simulink model "VFlexP_small"  (R2026a)
settings: Solver=ode23tb  StopTime=2  FixedStep=5e-5
model workspace (MAT data in the model file):
  DCop_DCBUCK : object (value not decoded)
  Grid_CCVSC_idx = [2; 3; 4; 5; 6; 7; 8; 9; 10; 11; 12]
  Grid_CCVSCs = 1
  Grid_CCVSCs_buses = 1
  Grid_CCVSCs_toM = [0 1 0 0 0 0 0 0 0 0 0 0 ... (781 elements, 71x11)]
  Grid_C_Lines = 0
  Grid_Cbuses = [0.00666666666667 0.00666666666667]
  Grid_DC : object (value not decoded)
  Grid_DCop_DCBUCK : object (value not decoded)
  Grid_DCop_DC_PES : object (value not decoded)
  Grid_DFIGs = 1
  Grid_DFIGs_buses = 1
  Grid_DGs : string (value not decoded)
  Grid_From_buses = 1
  Grid_GFls = 1
  Grid_GFls_buses = 1
  Grid_GFr_idx = 1
  Grid_GFrs = 1
  Grid_GFrs_buses = 1
  Grid_GFrs_toM = [1; 0]
  Grid_IG_idx = 1
  Grid_IGs = 1
  Grid_IGs_buses = 1
  Grid_IGs_toM = [1; 0; 0]
  Grid_L_Lines = 0.05
  Grid_L_Loads = [0 0]
  Grid_Lines_fromM : object (value not decoded)
  Grid_Lines_toM : object (value not decoded)
  Grid_Load_buses = [1; 2]
  Grid_Load_busesDC = []
  Grid_MSGs = 1
  Grid_MSGs_buses = 1
  Grid_Nbuses = 2
  Grid_PQ_gen = 3
  Grid_Ploads = [0.0075 0.0075]
  Grid_PloadsDC = []
  Grid_Ps_lf = 0.51232912
  Grid_Qloads = [0 0]
  Grid_Qs_lf = -0.00723209333333
  Grid_R_Lines = 0.005
  Grid_R_Loads = [2 2]
  Grid_R_Loads_DC = 0
  Grid_Rcf = [150 150]
  Grid_SCs = 1
  Grid_SCs_buses = 1
  Grid_SG_idx = 1
  Grid_SGs = 1
  Grid_SGs_buses = 1
  Grid_SGs_toM = [1; 0]
  Grid_To_buses = 2
  Grid_VCVSC_idx = [1; 2; 3; 4; 5; 6; 7; 8; 9; 10; 11; 12]
  Grid_VCVSCs = 1
  Grid_VCVSCs_buses = [1; 2; 3; 6; 8; 9; 12; 58; 59; 60; 63; 65]
  Grid_VCVSCs_toM = [1 0 0 0 0 0 0 0 0 0 0 0 ... (852 elements, 71x12)]
  Grid_VSM_idx = 2
  Grid_VSMs = 1
  Grid_VSMs_buses = 1
  Grid_VSMs_toM = [0; 1]
  Grid_admitt_matrix = [2.15353135314-19.7953135314i  -1.9801980198+19.801980198i; -1.9801980198+19.801980198i  2.15353135314-19.7953135314i]
  Grid_admitt_matrix_noloads = [1.98686468647-19.7953135314i  -1.9801980198+19.801980198i; -1.9801980198+19.801980198i  1.98686468647-19.7953135314i]
  Grid_bus = [1; 2]
  Grid_busDC_complexity = 1
  Grid_busDC_complexity_PF = 2
  Grid_bus_complexity = [1 1]
  Grid_bus_complexity_PF = [1 1]
  Grid_buses_lf = 1
  Grid_conductance_matrix = 0.00666666666667
  Grid_conductance_matrix_noloads = 0.00666666666667
  Grid_fref : object (value not decoded)
  Grid_gen_static_params : mBase (value not decoded)
  Grid_iPs_lf = 1.95187031336
  Grid_iQs_lf = -138.272551792
  Grid_iadmitt_matrix = [2.88165849328-0.0982918688642i  2.87905051706-0.123273862303i; 2.87905051706-0.123273862303i  2.88165849328-0.0982918688642i]
  Grid_iadmitt_matrix_noloads = [37.5012524798-37.4874983544i  37.4987475202-37.5125016456i; 37.4987475202-37.5125016456i  37.5012524798-37.4874983544i]
  Grid_iconductance_matrix = 150
  Grid_iconductance_matrix_noloads = 150
  Grid_init_OK_bool = 1
  Grid_intconv_PF : object (value not decoded)
  Grid_lf_op : op_report (value not decoded)
  Grid_lineDC_complexity = []
  Grid_lineDC_complexity_PF = []
  Grid_line_complexity = 1
  Grid_line_complexity_PF = 3
  Grid_loadDC_complexity = []
  Grid_loadDC_complexity_PF = []
  Grid_load_complexity = [3 3]
  Grid_load_complexity_PF = [4 4]
  Grid_opDC_CCVSC : object (value not decoded)
  Grid_opDC_VSM : object (value not decoded)
  Grid_opGFr : object (value not decoded)
  Grid_opVCVSC : object (value not decoded)
  Grid_op_CCVSC : object (value not decoded)
  Grid_op_IG : object (value not decoded)
  Grid_op_SG : object (value not decoded)
  Grid_op_VSM : object (value not decoded)
  Grid_shift_lines = 0
  Grid_tap_lines = 1
  Grid_v_buses_mod = [1 1]
  LinsysParamChangeStruct : Param1 (value not decoded)
  Lline = 0.01
  Rline = 1e-05
  linsys : object (value not decoded)
values from neighbouring files (symbols this model uses):
  block_idx = evalin(mdlWks, [bvarname Generators{i} '_idx'])    [fun_init_units_callback.m]
  Fb = areas    [fun_MATPOWER_to_Excel.m]
  Fi = evalin('base', get_param(block, 'Fi'))    [fun_init_GFr.m]    (also in fun_init_intconv_DC_VSM.m)
  Lf = evalin('base', get_param(block, 'Lf'))    [fun_init_GFr.m]    (also in fun_init_intconv_DC_VSM.m)
  Rf = evalin('base', get_param(block, 'Rf'))    [fun_init_GFr.m]    (also in fun_init_intconv_DC_VSM.m)
symbols that are objects in the model workspace (value not decoded): Grid_DCop_DC_PES, Grid_DCop_DCBUCK, Grid_op_CCVSC, Grid_op_IG, Grid_op_SG, Grid_op_VSM, Grid_opDC_CCVSC, Grid_opDC_VSM, Grid_opGFr, Grid_opVCVSC
undefined symbols (not defined in the file or in its folder): block_buses_DC, CCVSC_idx, Cf, costs, costs2, DFIGs_nodes, DiscIntNeverNeededParam, entity, From_nodes, grid_linsys, Grid_op_DFIG, Grid_op_DFIG_PQ, Grid_op_MSG, Grid_op_SC, Grid_op_VCVSC, Hv, initial_states_grid, Kic, Kiv, Kp_theta, Kp_w, Kpc, Kpv, last_send, Lc, m, Matrix_flux_to_i, mD, mp, MSGs_buses, Nbuses_DC, nq, op_VCVSC, Psche, Rc, rkq1, rkq2, SCs_buses, SCs_nodes, sec_control_structure, set_asked, set_DG_up, set_extra_satur, set_sending_cost, SGs_buses, SGs_nodes, Tf, To_nodes, VI_L, VI_R, WOF_Tf, xkq1, xkq2
libraries: simulink x1045, eeGeneralControl x12, eeTransforms x1, sl_discontinuities x1
(part 9 of 50)

== system VFlexP_small/Grid/Loadflow/Loads/dynamic ==
  v_in_d : Inport
  v_in_q : Inport  Port=2
  Gain1 : Gain  Gain=L_Loads(load_complexity_PF == 1)
  Gain2 : Gain  Gain=R_Loads(load_complexity_PF == 1)
  Gain3 : Gain  Gain=R_Loads(load_complexity_PF == 1)
  Gain4 : Gain  Gain=L_Loads(load_complexity_PF == 1)
  Gain5 : Gain  Gain=omegab./L_Loads(load_complexity_PF == 1)
  Gain7 : Gain  Gain=omegab./L_Loads(load_complexity_PF == 1)
  One : Constant  OutDataTypeStr=Inherit: Inherit via back propagation
  Product : Product
  Product1 : Product
  Selector : Selector  InputPortWidth=length(Load_buses)  IndexOptions=Index vector (dialog)  Indices=find(load_complexity_PF == 1)  OutputSizes=1
  Selector1 : Selector  InputPortWidth=length(Load_buses)  IndexOptions=Index vector (dialog)  Indices=find(load_complexity_PF == 1)  OutputSizes=1
  Sum4 : Sum  Inputs=+-|
  Sum5 : Sum  Inputs=|-+
  Sum6 : Sum  Inputs=|++
  Sum7 : Sum  Inputs=-+|
  Sum8 : Sum  Inputs=|+-
  Sum9 : Sum  Inputs=-+|
  Zero : Constant  Value=0  OutDataTypeStr=Inherit: Inherit via back propagation
  Zero1 : Constant  Value=0  OutDataTypeStr=Inherit: Inherit via back propagation
  i_d : Integrator  InitialCondition=0.1
  i_q : Integrator  InitialCondition=-0.1
  to_all_Loads : Subsystem
  to_all_Loads1 : Subsystem
  id : Outport
  iq : Outport  Port=2
  wires:
  v_in_q/1 -> Selector1/1  "v_in_q"
  v_in_d/1 -> Selector/1  "v_in_d"
  Gain2/1 -> Sum4/2
  i_d/1 -> Gain1/1, Gain2/1, to_all_Loads/1(In1)  "id"
  Sum6/1 -> Gain5/1
  One/1 -> Product1/1, Product/2  "omega"
  Gain5/1 -> i_d/1
  Product/1 -> Sum6/2
  Sum8/1 -> Gain7/1
  Sum4/1 -> Sum7/2
  Product1/1 -> Sum8/2
  Gain4/1 -> Product/1
  Sum7/1 -> Sum6/1
  Gain3/1 -> Sum5/1
  Sum5/1 -> Sum9/2
  Gain7/1 -> i_q/1
  i_q/1 -> to_all_Loads1/1(In1), Gain3/1, Gain4/1  "iq"
  Gain1/1 -> Product1/2
  Sum9/1 -> Sum8/1
  Zero/1 -> Sum7/1  "v_out_d"
  Zero1/1 -> Sum9/1  "v_out_q"
  to_all_Loads/1(id) -> id/1
  to_all_Loads1/1(id) -> iq/1
  Selector/1 -> Sum4/1
  Selector1/1 -> Sum5/2

== system VFlexP_small/Grid/Loadflow/Loads/dynamic PQ ==
  v_in_d : Inport
  v_in_q : Inport  Port=2
  Constant : Constant  Value=Ploads(load_complexity_PF == 5)/Sb  VectorParams1D=off
  Constant1 : Constant  Value=Qloads(load_complexity_PF == 5)/Sb  VectorParams1D=off
  Divide : Product  Inputs=*/
  Divide1 : Product  Inputs=*/
  Integrator : Integrator  InitialCondition=Ploads/Sb
  Integrator1 : Integrator  InitialCondition=-Qloads/Sb
  One1 : Constant  Value=eps  OutDataTypeStr=Inherit: Inherit via back propagation
  Product{,1..5} (6 alike) : Product
  Selector : Selector  InputPortWidth=length(Load_buses)  IndexOptions=Index vector (dialog)  Indices=find(load_complexity_PF == 5)  OutputSizes=1
  Selector1 : Selector  InputPortWidth=length(Load_buses)  IndexOptions=Index vector (dialog)  Indices=find(load_complexity_PF == 5)  OutputSizes=1
  Sum : Sum  Inputs=|++
  Sum1 : Sum  Inputs=|+-
  Sum2 : Sum  Inputs=|+-
  Sum3 : Sum  Inputs=|+-
  Sum4 : Sum  Inputs=|++
  Sum5 : Sum  Inputs=|++
  to_all_Loads : Subsystem
  to_all_Loads1 : Subsystem
  id : Outport
  iq : Outport  Port=2
  wires:
  Product1/1 -> Sum/2
  Product/1 -> Sum/1
  Constant/1 -> Product/1, Product2/1  "Prefnew"
  Product2/1 -> Sum1/1
  v_in_q/1 -> Selector1/1
  Product3/1 -> Sum1/2
  Product5/1 -> Sum4/2
  Constant1/1 -> Product3/1, Product1/2  "Qrefnew"
  Product4/1 -> Sum4/1
  Sum/1 -> Divide/1
  v_in_d/1 -> Selector/1
  Sum1/1 -> Divide1/1
  Sum5/1 -> Divide/2, Divide1/2
  Divide/1 -> Sum2/1  "idref"
  Sum2/1 -> Integrator/1
  Integrator/1 -> to_all_Loads/1(In1), Sum2/2
  Integrator1/1 -> to_all_Loads1/1(In1), Sum3/2
  Sum3/1 -> Integrator1/1
  Divide1/1 -> Sum3/1  "idref"
  Selector/1 -> Product4/1, Product4/2, Product/2, Product3/2
  to_all_Loads/1(Out1) -> id/1
  to_all_Loads1/1(Out1) -> iq/1
  Selector1/1 -> Product5/1, Product5/2, Product2/2, Product1/1
  Sum4/1 -> Sum5/1
  One1/1 -> Sum5/2

== system VFlexP_small/Grid/Loadflow/Loads/static ==
  v_in_d : Inport
  v_in_q : Inport  Port=2
  Constant : Constant  Value=R_Loads(load_complexity_PF == 2).^2  VectorParams1D=off
  Constant1 : Constant
  Divide : Product  Inputs=*/
  Gain : Gain  Gain=L_Loads(load_complexity_PF == 2)
  Gain1 : Gain  Gain=R_Loads(load_complexity_PF == 2)
  Gain2 : Gain  Gain=R_Loads(load_complexity_PF == 2)
  Product{,1..5} (6 alike) : Product
  Selector : Selector  InputPortWidth=length(Load_buses)  IndexOptions=Index vector (dialog)  Indices=find(load_complexity_PF == 2)  OutputSizes=1
  Selector1 : Selector  InputPortWidth=length(Load_buses)  IndexOptions=Index vector (dialog)  Indices=find(load_complexity_PF == 2)  OutputSizes=1
  Sum : Sum  Inputs=|++
  Sum1 : Sum  Inputs=|+-
  Sum2 : Sum  Inputs=|+-
  Sum3 : Sum  Inputs=|++
  Sum4 : Sum  Inputs=|-+
  Zero : Constant  Value=0  OutDataTypeStr=Inherit: Inherit via back propagation
  Zero1 : Constant  Value=0  OutDataTypeStr=Inherit: Inherit via back propagation
  to_all_Loads : Subsystem
  to_all_Loads1 : Subsystem
  id : Outport
  iq : Outport  Port=2
  wires:
  v_in_q/1 -> Selector1/1  "v_in_q"
  Zero/1 -> Sum1/2  "v_out_d"
  Sum/1 -> Divide/2
  Gain2/1 -> Product5/2
  Product/1 -> Sum/2
  Product1/1 -> Sum3/1
  Product5/1 -> Sum4/2
  Constant/1 -> Sum/1
  Sum2/1 -> Product3/2, Product5/1  "vq"
  Gain/1 -> Product2/2, Product/1, Product/2
  Constant1/1 -> Divide/1
  Product3/1 -> Sum3/2
  Sum1/1 -> Product4/1, Product1/1  "vd"
  Divide/1 -> Product2/1, Gain1/1, Gain2/1
  Product4/1 -> Sum4/1
  Product2/1 -> Product3/1, Product4/2
  Gain1/1 -> Product1/2
  Sum3/1 -> to_all_Loads/1(In1)  "id"
  Sum4/1 -> to_all_Loads1/1(In1)  "iq"
  Zero1/1 -> Sum2/2  "v_out_q"
  v_in_d/1 -> Selector/1  "v_in_d"
  [omega_ref] -> Gain/1  "omega"
  to_all_Loads/1(id) -> id/1
  to_all_Loads1/1(id) -> iq/1
  Selector/1 -> Sum1/1
  Selector1/1 -> Sum2/1

== system VFlexP_small/Grid/Loadflow/Loads/static omega ==
  v_in_d : Inport
  v_in_q : Inport  Port=2
  Gain : Gain  Gain=1./(R_Loads(load_complexity_PF == 3, :).^2+L_Loads(load_complexity_PF == 3, :).^2)
  Gain2 : Gain  Gain=1./(R_Loads(load_complexity_PF == 3, :).^2+L_Loads(load_complexity_PF == 3, :).^2)
  Gain3 : Gain  Gain=R_Loads(load_complexity_PF == 3, :)
  Gain4 : Gain  Gain=L_Loads(load_complexity_PF == 3, :)
  Gain5 : Gain  Gain=L_Loads(load_complexity_PF == 3, :)
  Gain6 : Gain  Gain=R_Loads(load_complexity_PF == 3, :)
  Selector : Selector  InputPortWidth=length(Load_buses)  IndexOptions=Index vector (dialog)  Indices=find(load_complexity_PF == 3)  OutputSizes=1
  Selector1 : Selector  InputPortWidth=length(Load_buses)  IndexOptions=Index vector (dialog)  Indices=find(load_complexity_PF == 3)  OutputSizes=1
  Sum : Sum  Inputs=|++
  Sum3 : Sum  Inputs=|-+
  to_all_Loads : Subsystem
  to_all_Loads1 : Subsystem
  id : Outport
  iq : Outport  Port=2
  wires:
  Gain6/1 -> Sum3/2
  Gain5/1 -> Sum3/1
  Gain2/1 -> Gain4/1, Gain6/1
  Gain4/1 -> Sum/2
  Gain3/1 -> Sum/1
  Gain/1 -> Gain3/1, Gain5/1
  v_in_d/1 -> Selector/1  "v_in_d"
  v_in_q/1 -> Selector1/1  "v_in_q"
  Sum/1 -> to_all_Loads/1(In1)
  Sum3/1 -> to_all_Loads1/1(In1)
  to_all_Loads/1(id) -> id/1
  Selector/1 -> Gain/1
  Selector1/1 -> Gain2/1
  to_all_Loads1/1(id) -> iq/1

== system VFlexP_small/Grid/Dynamic/DCAC converters/DC_CCVSC/CC ==
  note: 1) Add Subsystem or Model blocks as valid variant choices.
      | 2) You cannot connect blocks at this level. At simulation, connectivity is automatically
      | determined, based on the active variant and port name matching.
  idref : Inport
  iqref : Inport  Port=2
  vod : Inport  Port=3
  voq : Inport  Port=4
  omega : Inport  Port=5
  dynamic : Subsystem  VariantControl=dynamic  mask{dynamic_line=Dynamic}
      mask prompts: dynamic_line "Line"
      mask TypeOptions dynamic_line: RL/dynamic
  static : Subsystem  VariantControl=static
  idiref : Outport
  iqiref : Outport  Port=2
  vid : Outport  Port=3
  viq : Outport  Port=4

== system VFlexP_small/Grid/Dynamic/DCAC converters/DC_CCVSC/For Each Subsystem ==
  In1 : Inport  Partition=on  PartitionDimension=1  PartitionWidth=1  PartitionOffset=0
  For Each : ForEach  DisableCoverage=on
  State-Space : StateSpace  A=[]  B=[]  C=[]  D=block_toM  InitialCondition=0  ParameterTunability=Optimized
  Transpose : Math  Operator=transpose
  Transpose1 : Math  Operator=transpose
  Out1 : Outport  ConcatenationDimension=1
  wires:
  In1/1 -> Transpose/1
  Transpose1/1 -> Out1/1
  Transpose/1 -> State-Space/1
  State-Space/1 -> Transpose1/1

== system VFlexP_small/Grid/Dynamic/DCAC converters/DC_CCVSC/LPF_d ==
  In1 : Inport
  Gain : Gain  Gain=iTf
  I : Integrator  InitialCondition=Grid_opDC_CCVSC.P
  Sum4 : Sum  Inputs=|+-
  Out1 : Outport
  wires:
  Gain/1 -> I/1
  Sum4/1 -> Gain/1
  In1/1 -> Sum4/1
  I/1 -> Out1/1, Sum4/2

== system VFlexP_small/Grid/Dynamic/DCAC converters/DC_CCVSC/LPF_q ==
  In1 : Inport
  Gain : Gain  Gain=iTf
  I : Integrator  InitialCondition=Grid_opDC_CCVSC.Q
  Sum4 : Sum  Inputs=|+-
  Out1 : Outport
  wires:
  Gain/1 -> I/1
  I/1 -> Out1/1, Sum4/2
  In1/1 -> Sum4/1
  Sum4/1 -> Gain/1

== system VFlexP_small/Grid/Dynamic/DCAC converters/DC_CCVSC/PC ==
  vodi : Inport
  voq : Inport  Port=2
  vodi1 : Inport  Port=3
  vodi2 : Inport  Port=4
  omega : Inport  Port=5
  Constant : Constant
  Constant1 : Constant  Value=Eref  VectorParams1D=off
  Constant2 : Constant  Value=Inf
  Divide : Product  Inputs=*/
  Divide1 : Product  Inputs=*/
  Gain1 : Gain  Gain=alphaqcoef
  Gain2 : Gain  Gain=alphapcoef
  LPF_d : Subsystem
  LPF_q : Subsystem
  Product{,1..5} (6 alike) : Product
  Saturation : Subsystem  Commented=through
  Sum : Sum  Inputs=|++
  Sum1 : Sum  Inputs=|+-
  Sum3 : Sum  Inputs=|-+
  Sum4 : Sum  Inputs=|++
  Sum5 : Sum  Inputs=++|
  Sum6 : Sum  Inputs=|-+
  Sum7 : Sum  Inputs=++|
  Switch : Switch  Criteria=u2 > Threshold  Threshold=1e-5  ZeroCross=off  SaturateOnIntegerOverflow=off  InputSameDT=off
  Output : Outport
  Output1 : Outport  Port=2
  wires:
  Saturation/2(y1) -> Output1/1
  Saturation/1(y) -> Output/1
  Divide1/1 -> Saturation/2(ilqref)  "ilqref"
  Divide/1 -> Saturation/1(ildref)  "ildref"
  Product/1 -> Sum/1
  Product1/1 -> Sum/2
  Product2/1 -> Sum1/1
  Product3/1 -> Sum1/2
  Sum7/1 -> Product1/2, Product3/1  "Qrefnew"
  vodi/1 -> LPF_d/1(In1)  "vod"
  voq/1 -> LPF_q/1(In1)  "voq"
  Product4/1 -> Sum4/1
  Product5/1 -> Sum4/2
  Sum5/1 -> Product2/1, Product/1  "Prefnew"
  Sum1/1 -> Divide1/1
  Sum4/1 -> Switch/2, Switch/1
  Sum/1 -> Divide/1
  Sum3/1 -> Gain2/1
  Constant/1 -> Sum3/2
  Gain2/1 -> Sum5/1
  vodi1/1 -> Sum5/2  "Pref"
  Constant1/1 -> Sum6/2
  Gain1/1 -> Sum7/1
  omega/1 -> Sum3/1  "omega"
  Sum6/1 -> Gain1/1
  vodi2/1 -> Sum7/2  "Qref"
  Constant2/1 -> Switch/3
  Switch/1 -> Divide/2, Divide1/2
  LPF_d/1(Out1) -> Sum6/1, Product3/2, Product/2, Product4/2, Product4/1
  LPF_q/1(Out1) -> Product1/1, Product2/2, Product5/2, Product5/1

== system VFlexP_small/Grid/Dynamic/DCAC converters/DC_CCVSC/PLL ==
  note: 1) Add Subsystem or Model blocks as valid variant choices.
      | 2) You cannot connect blocks at this level. At simulation, connectivity is automatically
      | determined, based on the active variant and port name matching.
  voutangle : Inport
  vq : Inport  Port=2
  omega : Inport  Port=3
  dynamic : Subsystem  VariantControl=dynamic
  static : Subsystem  VariantControl=static
  theta : Outport
  omega_point : Outport  Port=2

== system VFlexP_small/Grid/Dynamic/DCAC converters/DC_CCVSC/Reference frame transform3 ==
  in_d : Inport
  theta : Inport  Port=2
  in_q : Inport  Port=3
  Complex to Real-Imag : ComplexToRealImag
  Cos : Trigonometry  SCDEnableBlockLinearizationSpecification=on  Operator=cos
  Product : Product
  Real-Imag to Complex : RealImagToComplex
  Real-Imag to Complex1 : RealImagToComplex
  Sin : Trigonometry  SCDEnableBlockLinearizationSpecification=on
  out_d : Outport
  out_q : Outport  Port=2
  wires:
  in_d/1 -> Real-Imag to Complex/1
  in_q/1 -> Real-Imag to Complex/2
  Complex to Real-Imag/1 -> out_d/1
  Sin/1 -> Real-Imag to Complex1/2
  Cos/1 -> Real-Imag to Complex1/1
  theta/1 -> Cos/1, Sin/1
  Product/1 -> Complex to Real-Imag/1
  Real-Imag to Complex/1 -> Product/2
  Real-Imag to Complex1/1 -> Product/1
  Complex to Real-Imag/2 -> out_q/1

== system VFlexP_small/Grid/Dynamic/DCAC converters/DC_CCVSC/Reference_frame_transform1 ==
  din : Inport
  qin : Inport  Port=2
  theta : Inport  Port=3
  Complex to Real-Imag : ComplexToRealImag
  Cos : Trigonometry  SCDEnableBlockLinearizationSpecification=on  Operator=cos
  Product : Product
  Real-Imag to Complex : RealImagToComplex
  Real-Imag to Complex1 : RealImagToComplex
  Sin : Trigonometry  SCDEnableBlockLinearizationSpecification=on
  dout : Outport
  qout : Outport  Port=2
  wires:
  Complex to Real-Imag/1 -> dout/1
  Complex to Real-Imag/2 -> qout/1
  Real-Imag to Complex1/1 -> Product/1
  din/1 -> Real-Imag to Complex/1
  qin/1 -> Real-Imag to Complex/2
  Real-Imag to Complex/1 -> Product/2
  Product/1 -> Complex to Real-Imag/1
  theta/1 -> Sin/1, Cos/1
  Cos/1 -> Real-Imag to Complex1/1
  Sin/1 -> Real-Imag to Complex1/2

== system VFlexP_small/Grid/Dynamic/DCAC converters/DC_CCVSC/connect ==
  id : Inport
  iq : Inport  Port=2
  connect : Inport  Port=3
  Switch : Switch  Criteria=u2 > Threshold  ZeroCross=off  SaturateOnIntegerOverflow=off  InputSameDT=off
  Switch1 : Switch  Criteria=u2 > Threshold  ZeroCross=off  SaturateOnIntegerOverflow=off  InputSameDT=off
  Zero1 : Constant  Value=0  VectorParams1D=off  OutDataTypeStr=Inherit: Inherit via back propagation
  Zero2 : Constant  Value=0  VectorParams1D=off  OutDataTypeStr=Inherit: Inherit via back propagation
  id_real : Outport
  iq_real : Outport  Port=2
  connected : Outport  Port=3  OutDataTypeStr=boolean
  wires:
  Zero2/1 -> Switch1/3
  iq/1 -> Switch1/1
  Switch1/1 -> iq_real/1
  connect/1 -> Switch/2, Switch1/2, connected/1
  id/1 -> Switch/1
  Zero1/1 -> Switch/3
  Switch/1 -> id_real/1

== system VFlexP_small/Grid/Dynamic/DCAC converters/DC_CCVSC/connect1 ==
  id : Inport
  iq : Inport  Port=2
  connect : Inport  Port=3
  Switch : Switch  Criteria=u2 > Threshold  ZeroCross=off  SaturateOnIntegerOverflow=off  InputSameDT=off
  Switch1 : Switch  Criteria=u2 > Threshold  ZeroCross=off  SaturateOnIntegerOverflow=off  InputSameDT=off
  Zero1 : Constant  Value=0  VectorParams1D=off  OutDataTypeStr=Inherit: Inherit via back propagation
  Zero2 : Constant  Value=0  VectorParams1D=off  OutDataTypeStr=Inherit: Inherit via back propagation
  id_real : Outport
  iq_real : Outport  Port=2
  wires:
  Switch/1 -> id_real/1
  Zero1/1 -> Switch/3
  id/1 -> Switch/1
  connect/1 -> Switch1/2, Switch/2
  Switch1/1 -> iq_real/1
  iq/1 -> Switch1/1
  Zero2/1 -> Switch1/3

== system VFlexP_small/Grid/Dynamic/DCAC converters/DC_CCVSC/trim_output ==
  id : Inport
  iq : Inport  Port=2
  vd : Inport  Port=3
  vq : Inport  Port=4
  Out1 : Outport
  Out2 : Outport  Port=2
  Out3 : Outport  Port=3
  Out4 : Outport  Port=4
  wires:
  iq/1 -> Out2/1
  vd/1 -> Out3/1
  vq/1 -> Out4/1
  id/1 -> Out1/1

== system VFlexP_small/Grid/Dynamic/DCAC converters/DC_VCVSC/For Each Subsystem ==
  In1 : Inport  Partition=on  PartitionDimension=1  PartitionWidth=1  PartitionOffset=0
  For Each : ForEach  DisableCoverage=on
  State-Space : StateSpace  A=[]  B=[]  C=[]  D=block_toM  InitialCondition=0  ParameterTunability=Optimized
  Transpose : Math  Operator=transpose
  Transpose1 : Math  Operator=transpose
  Out1 : Outport  ConcatenationDimension=1
  wires:
  In1/1 -> Transpose/1
  Transpose1/1 -> Out1/1
  Transpose/1 -> State-Space/1
  State-Space/1 -> Transpose1/1

== system VFlexP_small/Grid/Dynamic/DCAC converters/DC_VCVSC/LPF ==
  In1 : Inport
  Gain : Gain  Gain=1e2
  I : Integrator  InitialCondition=Grid_op_VCVSC.op.States(4).x'
  Sum4 : Sum  Inputs=|+-
  Out1 : Outport
  wires:
  I/1 -> Sum4/2, Out1/1
  In1/1 -> Sum4/1
  Sum4/1 -> Gain/1
  Gain/1 -> I/1

== system VFlexP_small/Grid/Dynamic/DCAC converters/DC_VCVSC/LPF1 ==
  In1 : Inport
  Gain : Gain  Gain=1e2
  I : Integrator  InitialCondition=Grid_op_VCVSC.op.States(5).x'
  Sum4 : Sum  Inputs=|+-
  Out1 : Outport
  wires:
  Gain/1 -> I/1
  Sum4/1 -> Gain/1
  In1/1 -> Sum4/1
  I/1 -> Out1/1, Sum4/2

== system VFlexP_small/Grid/Dynamic/DCAC converters/DC_VCVSC/LPF2 ==
  In1 : Inport
  Gain : Gain  Gain=1e2
  I : Integrator  InitialCondition=Grid_op_VCVSC.States(3,:)
  Sum4 : Sum  Inputs=|+-
  Out1 : Outport
  wires:
  Gain/1 -> I/1
  Sum4/1 -> Gain/1
  In1/1 -> Sum4/1
  I/1 -> Out1/1, Sum4/2

== system VFlexP_small/Grid/Dynamic/DCAC converters/DC_VCVSC/LPF3 ==
  In1 : Inport
  Gain : Gain  Gain=1e2
  I : Integrator  InitialCondition=Grid_op_VCVSC.States(4,:)
  Sum4 : Sum  Inputs=|+-
  Out1 : Outport
  wires:
  I/1 -> Sum4/2, Out1/1
  In1/1 -> Sum4/1
  Sum4/1 -> Gain/1
  Gain/1 -> I/1

== system VFlexP_small/Grid/Dynamic/DCAC converters/DC_VCVSC/PC ==
  ioq : Inport
  iodi : Inport  Port=2
  omegaref : Inport  Port=3
  Eref : Inport  Port=4
  vodi : Inport  Port=5
  voq : Inport  Port=6
  Psp : Inport  Port=7
  Qsp : Inport  Port=8
  LPF_P : Subsystem
  LPF_Q : Subsystem
  Product{,1..3} (4 alike) : Product
  Sum : Sum  Inputs=|++
  Sum1 : Sum  Inputs=|-+
  Sum2 : Sum  Inputs=|+-
  Sum3 : Sum  Inputs=|-+
  Sum4 : Sum  Inputs=|+-
  Sum5 : Sum  Inputs=-+|
  mp1 : Gain  Gain=mp
  nq1 : Gain  Gain=nq
  Out1 : Outport
  Out2 : Outport  Port=2
  P_f : Outport  Port=3
  Q_f : Outport  Port=4
  wires:
  LPF_Q/1(Q_f) -> nq1/1
  LPF_P/1(P_f) -> mp1/1
  Sum3/1 -> Out2/1  "vodref"
  Sum5/1 -> LPF_P/1(P)
  Psp/1 -> Sum5/1
  Sum4/1 -> LPF_Q/1(Q)
  Qsp/1 -> Sum4/2
  ioq/1 -> Product1/2, Product2/2  "ioq"
  iodi/1 -> Product/2, Product3/2  "iod"
  voq/1 -> Product3/1, Product1/1  "voq"
  mp1/1 -> Sum2/2  "mpP"
  Sum1/1 -> Sum4/1, Q_f/1
  Sum/1 -> P_f/1, Sum5/2
  omegaref/1 -> Sum2/1  "omegaref"
  Eref/1 -> Sum3/2  "Eref"
  nq1/1 -> Sum3/1  "nqQ"
  Product3/1 -> Sum1/2
  Product2/1 -> Sum1/1
  Product1/1 -> Sum/2
  Product/1 -> Sum/1
  vodi/1 -> Product/1, Product2/1  "vod"
  Sum2/1 -> Out1/1  "omega"

== system VFlexP_small/Grid/Dynamic/DCAC converters/DC_VCVSC/PI ==
  In1 : Inport
  Gain : Gain  Gain=0.1
  Gain1 : Gain  Gain=0.2
  I : Integrator  InitialCondition=Grid_op_VCVSC.States(7,:)
  Sum10 : Sum  Inputs=|++
  Out1 : Outport
  wires:
  In1/1 -> Gain1/1, Gain/1
  Sum10/1 -> Out1/1
  Gain/1 -> Sum10/1
  I/1 -> Sum10/2
  Gain1/1 -> I/1

== system VFlexP_small/Grid/Dynamic/DCAC converters/DC_VCVSC/PI1 ==
  In1 : Inport
  Gain : Gain  Gain=0.1/100/pi
  Gain1 : Gain  Gain=0.2/100/pi
  I : Integrator  InitialCondition=Grid_op_VCVSC.States(8,:)
  Sum10 : Sum  Inputs=|++
  Out1 : Outport
  wires:
  Gain1/1 -> I/1
  I/1 -> Sum10/2
  Gain/1 -> Sum10/1
  Sum10/1 -> Out1/1
  In1/1 -> Gain/1, Gain1/1

== system VFlexP_small/Grid/Dynamic/DCAC converters/DC_VCVSC/RL out ==
  note: 1) Add Subsystem or Model blocks as valid variant choices.
      | 2) You cannot connect blocks at this level. At simulation, connectivity is automatically
      | determined, based on the active variant and port name matching.
  v_in_d : Inport
  v_out_d : Inport  Port=2
  v_in_q : Inport  Port=3
  v_out_q : Inport  Port=4
  dynamic : Subsystem  VariantControl=dynamic
  static : Subsystem  VariantControl=static
  static_omega : Subsystem  VariantControl=static_omega
  id : Outport
  iq : Outport  Port=2
  v_outd : Outport  Port=3
  v_outq : Outport  Port=4

== system VFlexP_small/Grid/Dynamic/DCAC converters/DC_VCVSC/Reference frame transform1 ==
  in_d : Inport
  theta : Inport  Port=2
  in_q : Inport  Port=3
  Complex to Real-Imag : ComplexToRealImag
  Cos : Trigonometry  SCDEnableBlockLinearizationSpecification=on  Operator=cos
  Product : Product
  Real-Imag to Complex : RealImagToComplex
  Real-Imag to Complex1 : RealImagToComplex
  Sin : Trigonometry  SCDEnableBlockLinearizationSpecification=on
  out_d : Outport
  out_q : Outport  Port=2
  wires:
  in_d/1 -> Real-Imag to Complex/1
  in_q/1 -> Real-Imag to Complex/2
  Complex to Real-Imag/1 -> out_d/1
  Sin/1 -> Real-Imag to Complex1/2
  Cos/1 -> Real-Imag to Complex1/1
  theta/1 -> Cos/1, Sin/1
  Product/1 -> Complex to Real-Imag/1
  Real-Imag to Complex/1 -> Product/2
  Real-Imag to Complex1/1 -> Product/1
  Complex to Real-Imag/2 -> out_q/1

== system VFlexP_small/Grid/Dynamic/DCAC converters/DC_VCVSC/Reference frame transform2 ==
  in_d : Inport
  theta : Inport  Port=2
  in_q : Inport  Port=3
  Complex to Real-Imag : ComplexToRealImag
  Cos : Trigonometry  SCDEnableBlockLinearizationSpecification=on  Operator=cos
  Product : Product
  Real-Imag to Complex : RealImagToComplex
  Real-Imag to Complex1 : RealImagToComplex
  Sin : Trigonometry  SCDEnableBlockLinearizationSpecification=on
  out_d : Outport
  out_q : Outport  Port=2
  wires:
  Complex to Real-Imag/2 -> out_q/1
  Real-Imag to Complex1/1 -> Product/1
  Real-Imag to Complex/1 -> Product/2
  Product/1 -> Complex to Real-Imag/1
  theta/1 -> Sin/1, Cos/1
  Cos/1 -> Real-Imag to Complex1/1
  Sin/1 -> Real-Imag to Complex1/2
  Complex to Real-Imag/1 -> out_d/1
  in_q/1 -> Real-Imag to Complex/2
  in_d/1 -> Real-Imag to Complex/1

== system VFlexP_small/Grid/Dynamic/DCAC converters/DC_VCVSC/Reference frame transform3 ==
  in_d : Inport
  theta : Inport  Port=2
  in_q : Inport  Port=3
  Complex to Real-Imag : ComplexToRealImag
  Cos : Trigonometry  SCDEnableBlockLinearizationSpecification=on  Operator=cos
  Product : Product
  Real-Imag to Complex : RealImagToComplex
  Real-Imag to Complex1 : RealImagToComplex
  Sin : Trigonometry  SCDEnableBlockLinearizationSpecification=on
  out_d : Outport
  out_q : Outport  Port=2
  wires:
  in_d/1 -> Real-Imag to Complex/1
  in_q/1 -> Real-Imag to Complex/2
  Complex to Real-Imag/1 -> out_d/1
  Sin/1 -> Real-Imag to Complex1/2
  Cos/1 -> Real-Imag to Complex1/1
  theta/1 -> Sin/1, Cos/1
  Product/1 -> Complex to Real-Imag/1
  Real-Imag to Complex/1 -> Product/2
  Real-Imag to Complex1/1 -> Product/1
  Complex to Real-Imag/2 -> out_q/1

== system VFlexP_small/Grid/Dynamic/DCAC converters/DC_VCVSC/VCC ==
  note: 1) Add Subsystem or Model blocks as valid variant choices.
      | 2) You cannot connect blocks at this level. At simulation, connectivity is automatically
      | determined, based on the active variant and port name matching.
  vodref : Inport
  voqref : Inport  Port=2
  iod : Inport  Port=3
  ioq : Inport  Port=4
  omega : Inport  Port=5
  dynamic : Subsystem  VariantControl=dynamic
  dynamic_VC : Subsystem  VariantControl=dynamic_VC
  dynamic_limiting : Subsystem  VariantControl=dynamic_limiting
  static : Subsystem  VariantControl=static
  vidref : Outport
  viqref : Outport  Port=2

== system VFlexP_small/Grid/Dynamic/DCAC converters/DC_VCVSC/VI ==
  id : Inport
  iq : Inport  Port=2
  omega : Inport  Port=3
  Gain : Gain  Gain=L
  Gain1 : Gain  Gain=R
  Gain2 : Gain  Gain=L
  Gain3 : Gain  Gain=R
  Product : Product
  Product1 : Product
  Sum : Sum  Inputs=-+|
  Sum1 : Sum  Inputs=|--
  WOF_d : Subsystem  Commented=through
  WOF_q : Subsystem  Commented=through
  vd : Outport
  vq : Outport  Port=2
  wires:
  Gain/1 -> Product/1
  omega/1 -> Product/2, Product1/1
  iq/1 -> WOF_q/1(In1)
  Product/1 -> Sum/2
  id/1 -> WOF_d/1(In1)
  Gain2/1 -> Product1/2
  Product1/1 -> Sum1/1
  Gain1/1 -> Sum/1
  Gain3/1 -> Sum1/2
  Sum/1 -> vd/1
  Sum1/1 -> vq/1
  WOF_d/1(Out1) -> Gain2/1, Gain1/1
  WOF_q/1(Out1) -> Gain3/1, Gain/1

== system VFlexP_small/Grid/Dynamic/DCAC converters/DC_VCVSC/connect ==
  id : Inport
  iq : Inport  Port=2
  connect : Inport  Port=3
  Switch : Switch  Criteria=u2 > Threshold  ZeroCross=off  SaturateOnIntegerOverflow=off  InputSameDT=off
  Switch1 : Switch  Criteria=u2 > Threshold  ZeroCross=off  SaturateOnIntegerOverflow=off  InputSameDT=off
  Zero1 : Constant  Value=0  VectorParams1D=off  OutDataTypeStr=Inherit: Inherit via back propagation
  Zero2 : Constant  Value=0  VectorParams1D=off  OutDataTypeStr=Inherit: Inherit via back propagation
  id_real : Outport
  iq_real : Outport  Port=2
  connected : Outport  Port=3  OutDataTypeStr=boolean
  wires:
  Zero2/1 -> Switch1/3
  iq/1 -> Switch1/1
  Switch1/1 -> iq_real/1
  connect/1 -> Switch/2, Switch1/2, connected/1
  id/1 -> Switch/1
  Zero1/1 -> Switch/3
  Switch/1 -> id_real/1

== system VFlexP_small/Grid/Dynamic/DCAC converters/DC_VCVSC/trim_output ==
  id : Inport
  iq : Inport  Port=2
  vd : Inport  Port=3
  vq : Inport  Port=4
  Out1 : Outport
  Out2 : Outport  Port=2
  Out3 : Outport  Port=3
  Out4 : Outport  Port=4
  wires:
  iq/1 -> Out2/1
  vd/1 -> Out3/1
  vq/1 -> Out4/1
  id/1 -> Out1/1

== system VFlexP_small/Grid/Dynamic/DCAC converters/DC_VSM/For Each Subsystem ==
  In1 : Inport  Partition=on  PartitionDimension=1  PartitionWidth=1  PartitionOffset=0
  For Each : ForEach  DisableCoverage=on
  State-Space : StateSpace  A=[]  B=[]  C=[]  D=block_toM  InitialCondition=0  ParameterTunability=Optimized
  Transpose : Math  Operator=transpose
  Transpose1 : Math  Operator=transpose
  Out1 : Outport  ConcatenationDimension=1
  wires:
  State-Space/1 -> Transpose1/1
  Transpose/1 -> State-Space/1
  Transpose1/1 -> Out1/1
  In1/1 -> Transpose/1

== system VFlexP_small/Grid/Dynamic/DCAC converters/DC_VSM/LPF ==
  In1 : Inport
  Gain : Gain  Gain=1e2
  I : Integrator  InitialCondition=Grid_op_VCVSC.op.States(4).x'
  Sum4 : Sum  Inputs=|+-
  Out1 : Outport
  wires:
  Gain/1 -> I/1
  Sum4/1 -> Gain/1
  In1/1 -> Sum4/1
  I/1 -> Out1/1, Sum4/2

== system VFlexP_small/Grid/Dynamic/DCAC converters/DC_VSM/LPF1 ==
  In1 : Inport
  Gain : Gain  Gain=1e2
  I : Integrator  InitialCondition=Grid_op_VCVSC.op.States(5).x'
  Sum4 : Sum  Inputs=|+-
  Out1 : Outport
  wires:
  I/1 -> Sum4/2, Out1/1
  In1/1 -> Sum4/1
  Sum4/1 -> Gain/1
  Gain/1 -> I/1

== system VFlexP_small/Grid/Dynamic/DCAC converters/DC_VSM/LPF2 ==
  In1 : Inport
  Gain : Gain  Gain=10
  I : Integrator
  Sum4 : Sum  Inputs=|+-
  Out1 : Outport
  wires:
  I/1 -> Sum4/2, Out1/1
  In1/1 -> Sum4/1
  Sum4/1 -> Gain/1
  Gain/1 -> I/1

== system VFlexP_small/Grid/Dynamic/DCAC converters/DC_VSM/LPF_1 ==
  In1 : Inport
  Gain : Gain  Gain=6
  I : Integrator  InitialConditionSource=external  InitialCondition=Grid_op_VCVSC.op.States(6).x'
  Sum4 : Sum  Inputs=|+-
  Out1 : Outport
  wires:
  In1/1 -> Sum4/1, I/2
  Gain/1 -> I/1
  I/1 -> Out1/1, Sum4/2
  Sum4/1 -> Gain/1

== system VFlexP_small/Grid/Dynamic/DCAC converters/DC_VSM/LPF_2 ==
  In1 : Inport
  Gain : Gain  Gain=900
  I : Integrator  InitialConditionSource=external  InitialCondition=Grid_op_VCVSC.op.States(6).x'
  Sum4 : Sum  Inputs=|+-
  Out1 : Outport
  wires:
  Sum4/1 -> Gain/1
  I/1 -> Sum4/2, Out1/1
  Gain/1 -> I/1
  In1/1 -> I/2, Sum4/1

== system VFlexP_small/Grid/Dynamic/DCAC converters/DC_VSM/PC ==
  ioq : Inport
  iodi : Inport  Port=2
  omegaref : Inport  Port=3
  Eref : Inport  Port=4
  vodi : Inport  Port=5
  voq : Inport  Port=6
  Psp : Inport  Port=7
  Qsp : Inport  Port=8
  iomega : Inport  Port=9
  Divide : Product  Inputs=*/
  Gain : Gain  Gain=1./Rv
  Gain1 : Gain  Gain=Dv
  Gain2 : Gain  Gain=1./(2*Hv)
  IP : Integrator  InitialCondition=Grid_opDC_VSM.IP
  LPF_P : Subsystem
  LPF_P2 : Subsystem
  LPF_Q : Subsystem
  Product{,1..3} (4 alike) : Product
  Sum : Sum  Inputs=|++
  Sum1 : Sum  Inputs=|-+
  Sum2 : Sum  Inputs=|++
  Sum3 : Sum  Inputs=|-+
  Sum4 : Sum  Inputs=|+-
  Sum5 : Sum  Inputs=+|+|+
  Sum6 : Sum  Inputs=+-|
  Sum7 : Sum  Inputs=|+-
  Sum8 : Sum  Inputs=|+-
  Turbine model : Subsystem
  WOF_d : Subsystem
  nq1 : Gain  Gain=nq
  omega_i : Integrator  InitialCondition=1
  omega : Outport
  Out2 : Outport  Port=2
  P_f : Outport  Port=3
  Q_f : Outport  Port=4
  wires:
  vodi/1 -> Product2/1, Product/1  "vod"
  Product/1 -> Sum/1
  Product1/1 -> Sum/2
  Product2/1 -> Sum1/1
  Product3/1 -> Sum1/2
  nq1/1 -> Sum3/1  "nqQ"
  Eref/1 -> Sum3/2  "Eref"
  Sum1/1 -> Q_f/1, Sum4/1
  voq/1 -> Product1/1, Product3/1  "voq"
  iodi/1 -> Product3/2, Product/2  "iod"
  ioq/1 -> Product2/2, Product1/2  "ioq"
  Qsp/1 -> Sum4/2
  Sum4/1 -> LPF_Q/1(Q)
  Sum3/1 -> Out2/1  "vodref"
  LPF_Q/1(Q_f) -> nq1/1
  Gain2/1 -> omega_i/1
  Sum6/1 -> Gain/1
  Sum/1 -> Sum7/2, LPF_P2/1(P)
  omega_i/1 -> WOF_d/1(In1), Sum2/1, Sum6/2, Divide/2
  Gain/1 -> Sum5/1
  WOF_d/1(Out1) -> Gain1/1
  Turbine model/1(Out1) -> Sum7/1
  Gain1/1 -> Sum8/2
  Divide/1 -> Sum8/1
  Psp/1 -> Sum5/2
  Sum5/1 -> Turbine model/1(In1)
  Sum7/1 -> Divide/1
  Sum8/1 -> Gain2/1
  IP/1 -> Sum5/3
  omegaref/1 -> Sum6/1  "omegaref"
  Sum2/1 -> omega/1
  iomega/1 -> Sum2/2  "omegaref"
  LPF_P2/1(P_f) -> P_f/1

== system VFlexP_small/Grid/Dynamic/DCAC converters/DC_VSM/PLL ==
  out_q : Inport
  Gain : Gain  Gain=100
  Gain1 : Gain  Gain=1000
  I : Integrator
  Sum10 : Sum  Inputs=|++
  Input2 : Outport
  wires:
  Sum10/1 -> Input2/1
  out_q/1 -> Gain1/1, Gain/1
  Gain1/1 -> I/1
  Gain/1 -> Sum10/1
  I/1 -> Sum10/2

== system VFlexP_small/Grid/Dynamic/DCAC converters/DC_VSM/RL out ==
  note: 1) Add Subsystem or Model blocks as valid variant choices.
      | 2) You cannot connect blocks at this level. At simulation, connectivity is automatically
      | determined, based on the active variant and port name matching.
  v_in_d : Inport
  v_out_d : Inport  Port=2
  v_in_q : Inport  Port=3
  v_out_q : Inport  Port=4
  dynamic : Subsystem  VariantControl=dynamic
  static : Subsystem  VariantControl=static
  static_omega : Subsystem  VariantControl=static_omega
  id : Outport
  iq : Outport  Port=2
  v_outd : Outport  Port=3
  v_outq : Outport  Port=4

== system VFlexP_small/Grid/Dynamic/DCAC converters/DC_VSM/Reference frame transform1 ==
  in_d : Inport
  theta : Inport  Port=2
  in_q : Inport  Port=3
  Complex to Real-Imag : ComplexToRealImag
  Cos : Trigonometry  SCDEnableBlockLinearizationSpecification=on  Operator=cos
  Product : Product
  Real-Imag to Complex : RealImagToComplex
  Real-Imag to Complex1 : RealImagToComplex
  Sin : Trigonometry  SCDEnableBlockLinearizationSpecification=on
  out_d : Outport
  out_q : Outport  Port=2
  wires:
  Complex to Real-Imag/2 -> out_q/1
  Real-Imag to Complex1/1 -> Product/1
  Real-Imag to Complex/1 -> Product/2
  Product/1 -> Complex to Real-Imag/1
  theta/1 -> Sin/1, Cos/1
  Cos/1 -> Real-Imag to Complex1/1
  Sin/1 -> Real-Imag to Complex1/2
  Complex to Real-Imag/1 -> out_d/1
  in_q/1 -> Real-Imag to Complex/2
  in_d/1 -> Real-Imag to Complex/1

== system VFlexP_small/Grid/Dynamic/DCAC converters/DC_VSM/Reference frame transform2 ==
  in_d : Inport
  theta : Inport  Port=2
  in_q : Inport  Port=3
  Complex to Real-Imag : ComplexToRealImag
  Cos : Trigonometry  SCDEnableBlockLinearizationSpecification=on  Operator=cos
  Product : Product
  Real-Imag to Complex : RealImagToComplex
  Real-Imag to Complex1 : RealImagToComplex
  Sin : Trigonometry  SCDEnableBlockLinearizationSpecification=on
  out_d : Outport
  out_q : Outport  Port=2
  wires:
  in_d/1 -> Real-Imag to Complex/1
  in_q/1 -> Real-Imag to Complex/2
  Complex to Real-Imag/1 -> out_d/1
  Sin/1 -> Real-Imag to Complex1/2
  Cos/1 -> Real-Imag to Complex1/1
  theta/1 -> Cos/1, Sin/1
  Product/1 -> Complex to Real-Imag/1
  Real-Imag to Complex/1 -> Product/2
  Real-Imag to Complex1/1 -> Product/1
  Complex to Real-Imag/2 -> out_q/1

== system VFlexP_small/Grid/Dynamic/DCAC converters/DC_VSM/Reference frame transform3 ==
  in_d : Inport
  theta : Inport  Port=2
  in_q : Inport  Port=3
  Complex to Real-Imag : ComplexToRealImag
  Cos : Trigonometry  SCDEnableBlockLinearizationSpecification=on  Operator=cos
  Product : Product
  Real-Imag to Complex : RealImagToComplex
  Real-Imag to Complex1 : RealImagToComplex
  Sin : Trigonometry  SCDEnableBlockLinearizationSpecification=on
  out_d : Outport
  out_q : Outport  Port=2
  wires:
  Complex to Real-Imag/2 -> out_q/1
  Real-Imag to Complex1/1 -> Product/1
  Real-Imag to Complex/1 -> Product/2
  Product/1 -> Complex to Real-Imag/1
  theta/1 -> Cos/1, Sin/1
  Cos/1 -> Real-Imag to Complex1/1
  Sin/1 -> Real-Imag to Complex1/2
  Complex to Real-Imag/1 -> out_d/1
  in_q/1 -> Real-Imag to Complex/2
  in_d/1 -> Real-Imag to Complex/1

== system VFlexP_small/Grid/Dynamic/DCAC converters/DC_VSM/Reference frame transform4 ==
  in_d : Inport
  in_q : Inport  Port=2
  theta : Inport  Port=3
  Complex to Real-Imag : ComplexToRealImag
  Cos : Trigonometry  SCDEnableBlockLinearizationSpecification=on  Operator=cos
  Product : Product
  Real-Imag to Complex : RealImagToComplex
  Real-Imag to Complex1 : RealImagToComplex
  Sin : Trigonometry  SCDEnableBlockLinearizationSpecification=on
  out_d : Outport
  out_q : Outport  Port=2
  wires:
  Complex to Real-Imag/2 -> out_q/1
  Real-Imag to Complex1/1 -> Product/1
  Real-Imag to Complex/1 -> Product/2
  Product/1 -> Complex to Real-Imag/1
  theta/1 -> Sin/1, Cos/1
  Cos/1 -> Real-Imag to Complex1/1
  Sin/1 -> Real-Imag to Complex1/2
  Complex to Real-Imag/1 -> out_d/1
  in_q/1 -> Real-Imag to Complex/2
  in_d/1 -> Real-Imag to Complex/1

== system VFlexP_small/Grid/Dynamic/DCAC converters/DC_VSM/VCC ==
  note: 1) Add Subsystem or Model blocks as valid variant choices.
      | 2) You cannot connect blocks at this level. At simulation, connectivity is automatically
      | determined, based on the active variant and port name matching.
  vodref : Inport
  voqref : Inport  Port=2
  iod : Inport  Port=3
  ioq : Inport  Port=4
  omega : Inport  Port=5
  iP : Inport  Port=6
  dynamic : Subsystem  VariantControl=dynamic
  dynamic_VC : Subsystem  VariantControl=dynamic_VC
  dynamic_limiting : Subsystem  VariantControl=dynamic_limiting
  dynamic_limiting_P : Subsystem  VariantControl=dynamic_limiting_P
  static : Subsystem  VariantControl=static
  vidref : Outport
  viqref : Outport  Port=2
  iq_limited : Outport  Port=3
  iid : Outport  Port=4
  iiq : Outport  Port=5
  vid : Outport  Port=6
  viq : Outport  Port=7

== system VFlexP_small/Grid/Dynamic/DCAC converters/DC_VSM/VI ==
  id : Inport
  iq : Inport  Port=2
  omega : Inport  Port=3
  Gain : Gain  Gain=L
  Gain1 : Gain  Gain=R
  Gain2 : Gain  Gain=L
  Gain3 : Gain  Gain=R
  Product : Product
  Product1 : Product
  Sum : Sum  Inputs=-+|
  Sum1 : Sum  Inputs=|--
  WOF_d : Subsystem  Commented=through
  WOF_q : Subsystem  Commented=through
  vd : Outport
  vq : Outport  Port=2
  wires:
  WOF_q/1(Out1) -> Gain/1, Gain3/1
  WOF_d/1(Out1) -> Gain1/1, Gain2/1
  Sum1/1 -> vq/1
  Sum/1 -> vd/1
  Gain3/1 -> Sum1/2
  Gain1/1 -> Sum/1
  Product1/1 -> Sum1/1
  Gain2/1 -> Product1/2
  id/1 -> WOF_d/1(In1)
  Product/1 -> Sum/2
  iq/1 -> WOF_q/1(In1)
  omega/1 -> Product1/1, Product/2
  Gain/1 -> Product/1

== system VFlexP_small/Grid/Dynamic/DCAC converters/DC_VSM/WOF_d ==
  In1 : Inport
  Gain : Gain  Gain=100
  Gain1 : Gain  Gain=100
  I : Integrator  InitialConditionSource=external  InitialCondition=Grid_op_VCVSC.op.States(6).x'
  Sum : Sum  Inputs=+-|
  Sum4 : Sum  Inputs=|+-
  Out1 : Outport
  wires:
  Sum/1 -> Out1/1
  I/1 -> Sum4/2, Sum/2
  In1/1 -> Gain1/1
  Sum4/1 -> Gain/1
  Gain/1 -> I/1
  Gain1/1 -> I/2, Sum4/1, Sum/1

== system VFlexP_small/Grid/Dynamic/DCAC converters/DC_VSM/connect ==
  id : Inport
  iq : Inport  Port=2
  connect : Inport  Port=3
  Switch : Switch  Criteria=u2 > Threshold  ZeroCross=off  SaturateOnIntegerOverflow=off  InputSameDT=off
  Switch1 : Switch  Criteria=u2 > Threshold  ZeroCross=off  SaturateOnIntegerOverflow=off  InputSameDT=off
  Zero1 : Constant  Value=0  VectorParams1D=off  OutDataTypeStr=Inherit: Inherit via back propagation
  Zero2 : Constant  Value=0  VectorParams1D=off  OutDataTypeStr=Inherit: Inherit via back propagation
  id_real : Outport
  iq_real : Outport  Port=2
  connected : Outport  Port=3  OutDataTypeStr=boolean
  wires:
  Switch/1 -> id_real/1
  Zero1/1 -> Switch/3
  id/1 -> Switch/1
  connect/1 -> connected/1, Switch1/2, Switch/2
  Switch1/1 -> iq_real/1
  iq/1 -> Switch1/1
  Zero2/1 -> Switch1/3

== system VFlexP_small/Grid/Dynamic/DCAC converters/DC_VSM/trim_output ==
  id : Inport
  iq : Inport  Port=2
  vd : Inport  Port=3
  vq : Inport  Port=4
  Out1 : Outport
  Out2 : Outport  Port=2
  Out3 : Outport  Port=3
  Out4 : Outport  Port=4
  wires:
  id/1 -> Out1/1
  vq/1 -> Out4/1
  vd/1 -> Out3/1
  iq/1 -> Out2/1

== system VFlexP_small/Grid/Dynamic/Generators/DFIG/AVR_Vmeas_Filter ==
  in : Inport
  Gain : Gain  Gain=1/T_r
  Sum4 : Sum  Inputs=|+-
  x_a : Integrator  InitialCondition=Grid_op_DFIG.op.States(1).x'
  out : Outport
  wires:
  x_a/1 -> Sum4/2, out/1
  in/1 -> Sum4/1
  Sum4/1 -> Gain/1
  Gain/1 -> x_a/1

== system VFlexP_small/Grid/Dynamic/Generators/DFIG/AVR_Vmeas_Filter1 ==
  in : Inport
  Gain : Gain  Gain=1/T_r
  Sum4 : Sum  Inputs=|+-
  x_a : Integrator  InitialCondition=Grid_op_DFIG.op.States(2).x'
  out : Outport
  wires:
  Gain/1 -> x_a/1
  Sum4/1 -> Gain/1
  in/1 -> Sum4/1
  x_a/1 -> out/1, Sum4/2

== system VFlexP_small/Grid/Dynamic/Generators/DFIG/AVR_Vmeas_Filter2 ==
  in : Inport
  Gain : Gain  Gain=1/T_r
  Sum4 : Sum  Inputs=|+-
  x_a : Integrator  InitialCondition=Grid_op_DFIG.op.States(3).x'
  out : Outport
  wires:
  x_a/1 -> Sum4/2, out/1
  in/1 -> Sum4/1
  Sum4/1 -> Gain/1
  Gain/1 -> x_a/1

== system VFlexP_small/Grid/Dynamic/Generators/DFIG/Decoupling vrdqFs ==
  irq_Fs : Inport
  Vrd' : Inport  Port=2
  s : Inport  Port=3
  ws : Inport  Port=4
  ism : Inport  Port=5
  vrq' : Inport  Port=6
  ird_Fs : Inport  Port=7
  Subsystem1 : Subsystem
  Subsystem2 : Subsystem
  Sum : Sum  Inputs=|+-
  Sum1 : Sum  Inputs=|++
  vrd_Fs : Outport
  vrq_Fs : Outport  Port=2
  wires:
  vrq'/1 -> Sum1/1
  ird_Fs/1 -> Subsystem1/1(ird_Fs)
  irq_Fs/1 -> Subsystem2/1(irq_Fs)
  Sum/1 -> vrd_Fs/1
  Vrd'/1 -> Sum/1
  s/1 -> Subsystem2/2(s), Subsystem1/2(s)
  ws/1 -> Subsystem2/3(ws), Subsystem1/3(ws)
  Subsystem2/1(d) -> Sum/2
  Subsystem1/1(q) -> Sum1/2
  Sum1/1 -> vrq_Fs/1
  ism/1 -> Subsystem1/4(ism)

== system VFlexP_small/Grid/Dynamic/Generators/DFIG/For Each Subsystem ==
  In1 : Inport  Partition=on  PartitionDimension=1  PartitionWidth=1  PartitionOffset=0
  Assignment : Assignment  DiagnosticForDimensions=Warning  IndexOptions=Index vector (dialog)  Indices=block_buses  OutputSizes=1
  For Each : ForEach  DisableCoverage=on
  Zero : Constant  Value=zeros(1,Nbuses)  VectorParams1D=off  OutDataTypeStr=Inherit: Inherit via back propagation
  Out1 : Outport  ConcatenationDimension=1
  wires:
  Assignment/1 -> Out1/1
  In1/1 -> Assignment/2
  Zero/1 -> Assignment/1

== system VFlexP_small/Grid/Dynamic/Generators/DFIG/GSC Control ==
  vsd : Inport
  vsq : Inport  Port=2
  iad_ref : Inport  Port=3
  iad : Inport  Port=4
  iaq_ref : Inport  Port=5
  iaq : Inport  Port=6
  ws : Inport  Port=7
  PI Estator Current d : Subsystem
  PI Estator Current q : Subsystem
  Subsystem1 : Subsystem
  Subsystem3 : Subsystem
  Sum : Sum  Inputs=|+-
  Sum1 : Sum  Inputs=|+-
  vad : Outport  VectorParamsAs1DForOutWhenUnconnected=off
  vaq : Outport  Port=2  VectorParamsAs1DForOutWhenUnconnected=off
  wires:
  Subsystem1/1(vadq) -> vaq/1
  vsq/1 -> Subsystem1/3(vsq)
  ws/1 -> Subsystem3/4(ws), Subsystem1/1(ws)
  iaq/1 -> Sum1/2, Subsystem3/3(iaq)
  iaq_ref/1 -> Sum1/1
  iad_ref/1 -> Sum/1
  Sum/1 -> PI Estator Current d/1(in)
  Sum1/1 -> PI Estator Current q/1(in)
  iad/1 -> Subsystem1/4(iad), Sum/2
  PI Estator Current d/1(out) -> Subsystem3/1(vad')
  PI Estator Current q/1(out) -> Subsystem1/2(vaq')
  vsd/1 -> Subsystem3/2(vd)
  Subsystem3/1(vad) -> vad/1

== system VFlexP_small/Grid/Dynamic/Generators/DFIG/PI Q ==
  in : Inport
  Gain : Gain  Gain=0.25
  Gain1 : Gain  Gain=0.5
  Gain2 : Gain
  Gain3 : Gain
  Sum : Sum  Inputs=++|
  pi q : Integrator  InitialCondition=Grid_op_DFIG.op.States(8).x'  UpperSaturationLimit=1.01  LowerSaturationLimit=0.99
  out : Outport  VectorParamsAs1DForOutWhenUnconnected=off
  wires:
  pi q/1 -> Sum/2
  Gain/1 -> Gain2/1
  in/1 -> Gain/1, Gain1/1
  Sum/1 -> out/1
  Gain1/1 -> Gain3/1
  Gain2/1 -> Sum/1
  Gain3/1 -> pi q/1

== system VFlexP_small/Grid/Dynamic/Generators/DFIG/PI TE ==
  in : Inport
  Gain : Gain  Gain=0.25
  Gain1 : Gain  Gain=0.5
  Gain2 : Gain
  Gain3 : Gain
  Sum : Sum  Inputs=++|
  pi TE : Integrator  InitialCondition=Grid_op_DFIG.op.States(9).x'  UpperSaturationLimit=1.01  LowerSaturationLimit=0.99
  out : Outport  VectorParamsAs1DForOutWhenUnconnected=off
  wires:
  Gain1/1 -> Gain3/1
  Gain2/1 -> Sum/1
  Sum/1 -> out/1
  in/1 -> Gain1/1, Gain/1
  Gain/1 -> Gain2/1
  pi TE/1 -> Sum/2
  Gain3/1 -> pi TE/1

== system VFlexP_small/Grid/Dynamic/Generators/DFIG/PI v ==
  in : Inport
  Gain : Gain  Gain=0.25
  Gain1 : Gain  Gain=0.5
  Gain2 : Gain
  Gain3 : Gain
  Gain4 : Gain  Gain=0.000001
  Sum : Sum  Inputs=++|
  pi q : Integrator  InitialCondition=Grid_op_DFIG.op.States(10).x'  UpperSaturationLimit=1.01  LowerSaturationLimit=0.99
  out : Outport  VectorParamsAs1DForOutWhenUnconnected=off
  wires:
  Gain3/1 -> pi q/1
  Gain2/1 -> Sum/1
  Gain1/1 -> Gain3/1
  Sum/1 -> out/1
  in/1 -> Gain4/1
  Gain/1 -> Gain2/1
  pi q/1 -> Sum/2
  Gain4/1 -> Gain/1, Gain1/1

== system VFlexP_small/Grid/Dynamic/Generators/DFIG/PLL ==
  vdq0_meas : Inport
  Constant : Constant
  Gain1 : Gain  Gain=Ki_pll
  Gain2 : Gain  Gain=Kp_pll
  Gain4 : Gain  Gain=1/2/pi
  One1 : Constant  Value=0  OutDataTypeStr=Inherit: Inherit via back propagation
  Product1 : Product
  Product4 : Product
  Selector8 : Selector  InputPortWidth=length(fref.ref_units)  IndexOptions=Index vector (dialog)  Indices=block_fref  OutputSizes=1
  Sum : Sum  Inputs=|-+
  Sum1 : Sum  Inputs=|+-
  Sum2 : Sum  Inputs=++|
  dtheta_pll : Integrator  InitialCondition=Grid_op_DFIG.op.States(10).x'
  dw_pll : Integrator  InitialCondition=Grid_op_DFIG.op.States(11).x'
  theta_rad_pll : Outport
  omega_pu_pll : Outport  Port=2
  Freq_Hz_pll : Outport  Port=3
  wires:
  One1/1 -> Sum/1
  vdq0_meas/1 -> Sum/2
  Gain4/1 -> Freq_Hz_pll/1
  dw_pll/1 -> Sum2/2
  Gain2/1 -> Sum2/1
  Sum/1 -> Gain2/1, Gain1/1
  Gain1/1 -> dw_pll/1
  dtheta_pll/1 -> theta_rad_pll/1
  Product1/1 -> Gain4/1
  Sum2/1 -> Sum1/1, Product1/1, omega_pu_pll/1
  Sum1/1 -> Product4/1
  Constant/1 -> Sum1/2
  Product4/1 -> dtheta_pll/1
  Selector8/1 -> Product1/2, Product4/2
  [omega_base] -> Selector8/1

== system VFlexP_small/Grid/Dynamic/Generators/DFIG/RSC Control ==
  ird_Fs_ref : Inport
  ird_Fs_meas : Inport  Port=2
  irq_Fs_ref : Inport  Port=3
  irq_Fs_meas : Inport  Port=4
  PI Rotor Current d : Subsystem
  PI Rotor Current q : Subsystem
  Sum : Sum  Inputs=|+-
  Sum1 : Sum  Inputs=|+-
  vrd' : Outport  VectorParamsAs1DForOutWhenUnconnected=off
  vrq' : Outport  Port=2  VectorParamsAs1DForOutWhenUnconnected=off
  wires:
  Sum1/1 -> PI Rotor Current q/1(in)
  irq_Fs_ref/1 -> Sum1/1
  irq_Fs_meas/1 -> Sum1/2
  ird_Fs_meas/1 -> Sum/2
  PI Rotor Current q/1(out) -> vrq'/1
  PI Rotor Current d/1(out) -> vrd'/1
  Sum/1 -> PI Rotor Current d/1(in)
  ird_Fs_ref/1 -> Sum/1

== system VFlexP_small/Grid/Dynamic/Generators/DFIG/Reference frame transform2 ==
  vrd_Fs : Inport
  phi : Inport  Port=2
  vrq_Fs : Inport  Port=3
  Complex to Real-Imag : ComplexToRealImag
  Cos : Trigonometry  SCDEnableBlockLinearizationSpecification=on  Operator=cos
  Product : Product
  Real-Imag to Complex : RealImagToComplex
  Real-Imag to Complex1 : RealImagToComplex
  Sin : Trigonometry  SCDEnableBlockLinearizationSpecification=on
  vrd : Outport
  vrq : Outport  Port=2
  wires:
  Complex to Real-Imag/2 -> vrq/1
  Real-Imag to Complex1/1 -> Product/1
  Real-Imag to Complex/1 -> Product/2
  Product/1 -> Complex to Real-Imag/1
  phi/1 -> Sin/1, Cos/1
  Cos/1 -> Real-Imag to Complex1/1
  Sin/1 -> Real-Imag to Complex1/2
  Complex to Real-Imag/1 -> vrd/1
  vrq_Fs/1 -> Real-Imag to Complex/2
  vrd_Fs/1 -> Real-Imag to Complex/1

== system VFlexP_small/Grid/Dynamic/Generators/DFIG/Reference frame transform3 ==
  in_d : Inport
  theta : Inport  Port=2
  in_q : Inport  Port=3
  Complex to Real-Imag : ComplexToRealImag
  Cos : Trigonometry  SCDEnableBlockLinearizationSpecification=on  Operator=cos
  Product : Product
  Real-Imag to Complex : RealImagToComplex
  Real-Imag to Complex1 : RealImagToComplex
  Sin : Trigonometry  SCDEnableBlockLinearizationSpecification=on
  out_d : Outport
  out_q : Outport  Port=2
  wires:
  Complex to Real-Imag/2 -> out_q/1
  Real-Imag to Complex1/1 -> Product/1
  Real-Imag to Complex/1 -> Product/2
  Product/1 -> Complex to Real-Imag/1
  theta/1 -> Sin/1, Cos/1
  Cos/1 -> Real-Imag to Complex1/1
  Sin/1 -> Real-Imag to Complex1/2
  Complex to Real-Imag/1 -> out_d/1
  in_q/1 -> Real-Imag to Complex/2
  in_d/1 -> Real-Imag to Complex/1
